simulink model "DroneProjectFunctionalArchitecture"  (R2023b)
settings: Solver=VariableStepAuto  StartTime=0.0  StopTime=10.0  RelTol=1e-3
settings Model: Creator=carol  LastModifiedBy=carol

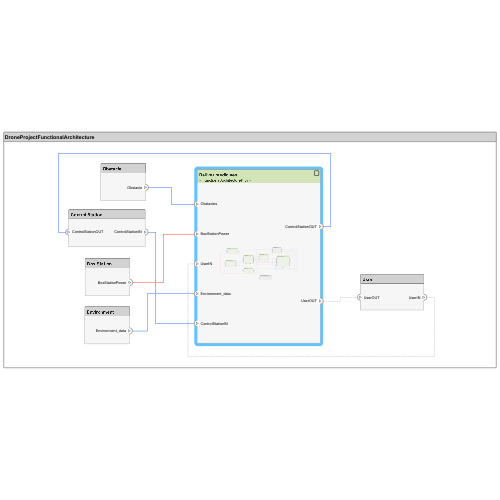
[thumbnail: Simulink's stored preview of the top-level diagram]
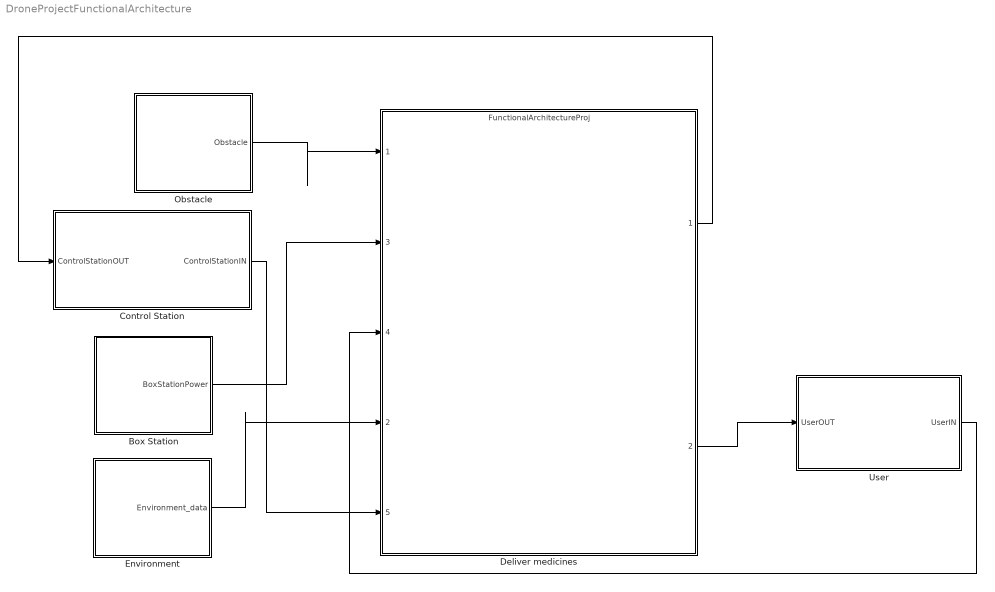
== system DroneProjectFunctionalArchitecture ==
  Box Station : Subsystem
      settings: PortSchema="{\"entries\":[{\"content\":{\"headerSize\":26,\"margin\":15,\"minimumSpacing\":25,\"sides\":[{\"content\":{},\"type\":\"ConnectorPlacement.EquallySpacedRectSide\",\"uuid\":\"4363930a-608c-49b3-a552-25912bab4631\"},{\"content\":{\"connectorIds\":[\"Out1\"],\"side\":\"RIGHT\"},\"type\":\"ConnectorPlacement.EquallySpacedRectSide\",\"uuid\":\"46b32956-08e1-442a-91b2-d83b199630ea\"},{\"content\":{\"side\":\"TOP\"},\"type\":\"ConnectorPlacement.EquallySpacedRectSide\",\"uuid\":\"ba364085-3ac2-4596-8832-357eb5446ff0\"}]},\"type\":\"ConnectorPlacement.EquallySpacedConnector\",\"uuid\":\"92fd45a1-4b9d-46f0-9585-9d2548d6ba77\"}],\"packageUris\":[\"http://schema.mathworks.com/mf0/Connector/R2020b\"],\"version\":\"1.0\"}"
  Control Station : Subsystem
      settings: PortSchema="{\"entries\":[{\"content\":{\"headerSize\":26,\"margin\":15,\"minimumSpacing\":25,\"sides\":[{\"content\":{\"connectorIds\":[\"In1\"]},\"type\":\"ConnectorPlacement.EquallySpacedRectSide\",\"uuid\":\"3b5ec35b-efef-42bc-989f-0358b373f88c\"},{\"content\":{\"connectorIds\":[\"Out1\"],\"side\":\"RIGHT\"},\"type\":\"ConnectorPlacement.EquallySpacedRectSide\",\"uuid\":\"39a24d49-19b9-4508-91cd-8aceba2ac1ea\"},{\"content\":{\"side\":\"TOP\"},\"type\":\"ConnectorPlacement.EquallySpacedRectSide\",\"uuid\":\"1edcc8ed-84b2-4c5f-810f-53183898c4f5\"}]},\"type\":\"ConnectorPlacement.EquallySpacedConnector\",\"uuid\":\"9d581d8a-2dea-49e6-903e-7a6990d5505f\"}],\"packageUris\":[\"http://schema.mathworks.com/mf0/Connector/R2020b\"],\"version\":\"1.0\"}"
  Deliver medicines : ModelReference  ModelNameDialog=FunctionalArchitectureProj  SimulationMode=Normal  ModelReferenceVersion=1.24
      settings: PortSchema="{\"entries\":[{\"content\":{\"headerSize\":38,\"margin\":15,\"minimumSpacing\":25,\"sides\":[{\"content\":{\"connectorIds\":[\"In1\",\"In3\",\"In4\",\"In2\",\"In5\"]},\"type\":\"ConnectorPlacement.EquallySpacedRectSide\",\"uuid\":\"3b5ec35b-efef-42bc-989f-0358b373f88c\"},{\"content\":{\"connectorIds\":[\"Out1\",\"Out2\"],\"side\":\"RIGHT\"},\"type\":\"ConnectorPlacement.EquallySpacedRectSide\",\"uuid\":\"39a24d49-19b9-4508-91cd-8aceba2ac1ea\"},{\"content\":{\"side\":\"TOP\"},\"type\":\"ConnectorPlacement.EquallySpacedRectSide\",\"uuid\":\"1edcc8ed-84b2-4c5f-810f-53183898c4f5\"},{\"content\":{\"side\":\"BOTTOM\"},\"type\":\"ConnectorPlacement.EquallySpacedRectSide\",\"uuid\":\"80d2382e-20f2-4450-b0cf-96f7ac15d2e4\"}]},\"type\":\"ConnectorPlacement.EquallySpacedConnector\",\"uuid\":\"9d581d8a-2dea-49e6-903e-7a6990d5505f\"}],\"packageUris\":[\"http://schema.mathworks.com/mf0/Connector/R2020b\"],\"version\":\"1.0\"}"
  Environment : Subsystem
      settings: PortSchema="{\"entries\":[{\"content\":{\"headerSize\":26,\"margin\":15,\"minimumSpacing\":25,\"sides\":[{\"content\":{},\"type\":\"ConnectorPlacement.EquallySpacedRectSide\",\"uuid\":\"3b5ec35b-efef-42bc-989f-0358b373f88c\"},{\"content\":{\"connectorIds\":[\"Out1\"],\"side\":\"RIGHT\"},\"type\":\"ConnectorPlacement.EquallySpacedRectSide\",\"uuid\":\"39a24d49-19b9-4508-91cd-8aceba2ac1ea\"},{\"content\":{\"side\":\"TOP\"},\"type\":\"ConnectorPlacement.EquallySpacedRectSide\",\"uuid\":\"1edcc8ed-84b2-4c5f-810f-53183898c4f5\"}]},\"type\":\"ConnectorPlacement.EquallySpacedConnector\",\"uuid\":\"9d581d8a-2dea-49e6-903e-7a6990d5505f\"}],\"packageUris\":[\"http://schema.mathworks.com/mf0/Connector/R2020b\"],\"version\":\"1.0\"}"
  Obstacle : Subsystem
      settings: PortSchema="{\"entries\":[{\"content\":{\"headerSize\":26,\"margin\":15,\"minimumSpacing\":25,\"sides\":[{\"content\":{},\"type\":\"ConnectorPlacement.EquallySpacedRectSide\",\"uuid\":\"4363930a-608c-49b3-a552-25912bab4631\"},{\"content\":{\"connectorIds\":[\"Out1\"],\"side\":\"RIGHT\"},\"type\":\"ConnectorPlacement.EquallySpacedRectSide\",\"uuid\":\"46b32956-08e1-442a-91b2-d83b199630ea\"},{\"content\":{\"side\":\"TOP\"},\"type\":\"ConnectorPlacement.EquallySpacedRectSide\",\"uuid\":\"ba364085-3ac2-4596-8832-357eb5446ff0\"}]},\"type\":\"ConnectorPlacement.EquallySpacedConnector\",\"uuid\":\"92fd45a1-4b9d-46f0-9585-9d2548d6ba77\"}],\"packageUris\":[\"http://schema.mathworks.com/mf0/Connector/R2020b\"],\"version\":\"1.0\"}"
  User : Subsystem
      settings: PortSchema="{\"entries\":[{\"content\":{\"headerSize\":26,\"margin\":15,\"minimumSpacing\":25,\"sides\":[{\"content\":{\"connectorIds\":[\"In1\"]},\"type\":\"ConnectorPlacement.EquallySpacedRectSide\",\"uuid\":\"4363930a-608c-49b3-a552-25912bab4631\"},{\"content\":{\"connectorIds\":[\"Out1\"],\"side\":\"RIGHT\"},\"type\":\"ConnectorPlacement.EquallySpacedRectSide\",\"uuid\":\"46b32956-08e1-442a-91b2-d83b199630ea\"},{\"content\":{\"side\":\"TOP\"},\"type\":\"ConnectorPlacement.EquallySpacedRectSide\",\"uuid\":\"ba364085-3ac2-4596-8832-357eb5446ff0\"}]},\"type\":\"ConnectorPlacement.EquallySpacedConnector\",\"uuid\":\"92fd45a1-4b9d-46f0-9585-9d2548d6ba77\"}],\"packageUris\":[\"http://schema.mathworks.com/mf0/Connector/R2020b\"],\"version\":\"1.0\"}"
  wires:
  Obstacle/1(Obstacle) -> Deliver medicines/1
  Environment/1(Environment_data) -> Deliver medicines/2
  Deliver medicines/1 -> Control Station/1(ControlStationOUT)
  Deliver medicines/2 -> User/1(UserOUT)
  User/1(UserIN) -> Deliver medicines/4
  Box Station/1(BoxStationPower) -> Deliver medicines/3
  Control Station/1(ControlStationIN) -> Deliver medicines/5

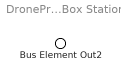
== system DroneProjectFunctionalArchitecture/Box Station ==
  Bus Element Out2 : Outport  PortName=BoxStationPower

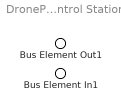
== system DroneProjectFunctionalArchitecture/Control Station ==
  Bus Element In1 : Inport  PortName=ControlStationOUT
  Bus Element Out1 : Outport  PortName=ControlStationIN

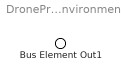
== system DroneProjectFunctionalArchitecture/Environment ==
  Bus Element Out1 : Outport  PortName=Environment_data

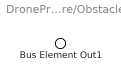
== system DroneProjectFunctionalArchitecture/Obstacle ==
  Bus Element Out1 : Outport  PortName=Obstacle

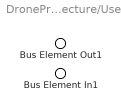
== system DroneProjectFunctionalArchitecture/User ==
  Bus Element In1 : Inport  PortName=UserOUT
  Bus Element Out1 : Outport  PortName=UserIN
